simulink library "CreeksideLibrary030"  (R2016b)
settings: Solver=VariableStepAuto  StartTime=0.0  StopTime=10.0  RelTol=1e-3  EnableMultiTasking=on
libraries: simulink x4
settings Model: Creator=Jared  LastModifiedBy=Ika
settings DataIOCC: LimitDataPoints=on
settings OptimizationCC: LifeSpan=inf
settings DebuggingCC: AllowSymbolicDim=off  SFUnexpectedBacktrackingDiag=warning  SFNoUnconditionalDefaultTransitionDiag=warning  SFExecutionAtInitializationDiag=none
settings ModelReferenceCC: PropagateSignalLabelsOutOfModel=off
settings GRTTargetCC: TargetLangStandard=C89/C90 (ANSI)
settings ConfigComp: CovMetricSettings=dw  CovHtmlReporting=on  CovSaveCumulativeToWorkspaceVar=on  CovSaveSingleToWorkspaceVar=on  CovExternalEMLEnable=off

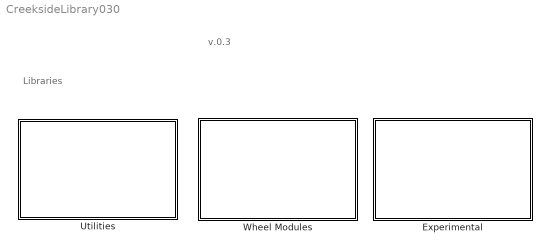
== system CreeksideLibrary030 ==
  note: Libraries
  note: v.0.3
  Experimental : Subsystem
      mask Display: image('gearBlock.png');
  Utilities : Subsystem
      mask Display: image('utilities.png');
  Wheel Modules : Subsystem
      mask Display: image('gearBlock.png');

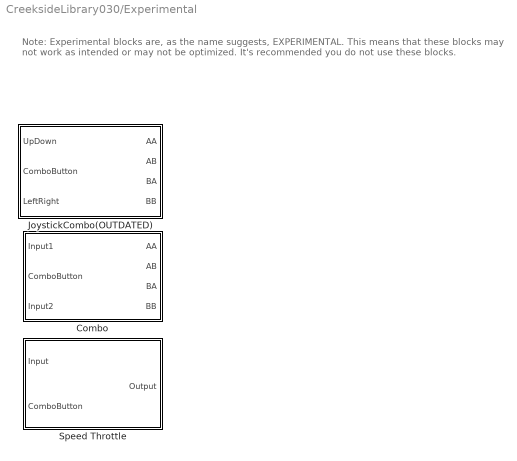
== system CreeksideLibrary030/Experimental ==
  note: Note: Experimental blocks are, as the name suggests, EXPERIMENTAL.
      | This means that these blocks may not work as intended or may not be optimized.
      | It's recommended you do not use these blocks.
  Combo : Subsystem  mask(Joystick Combo v.0.2.1){AAGain=1, ABGain=1, BAGain=1, BBGain=1}
      mask prompts: AAGain "AA value multiplier"; ABGain "AB value multiplier"; BAGain "BA value multiplier"; BBGain "BB value multiplier"
      mask help:
      | WARNING: Experimental version of Combo. This will have limited
      | functionality and may be buggy.
      |
      | Allows you to control multiple blocks using a joystick and a button.
      |
      | Link vertical joystick channels to UpDown, link horizontal joystick
      | channels LeftRight, and link a button to ComboButton.
      |
      | AA = Up/Down while not holding combo
      | AB = Left/Right while not holding combo
      | BA = Up/Down while holding combo
      | BB = Left/Right while holding combo
      mask Display:
      | pic = imread('globeMotor.png');
      | image(pic,[0.25 0.2 0.5 0.5]);
      | color('blue');
      | text(1,1,'CT','horizontalAlignment','right','verticalAlignment','top');
  JoystickCombo(OUTDATED) : MATLAB Function  TreatAsAtomicUnit=on  mask(Joystick Combo v.0.1.1){ButtonJoystick=off}
      mask prompts: ButtonJoystick "Using buttons?"
      mask help:
      | WARNING: Experimental version of Combo. This will have limited
      | functionality and may be buggy. Parameters have no effect on the block.
      |
      | Allows you to control multiple blocks using a joystick and a button.
      | Link vertical joystick channels to UpDown, link horizontal joystick
      | channels LeftRight, and link a button to ComboButton.
      |
      | AA = Up/Down while not holding combo
      | AB = Left/Right while not holding combo
      | BA = Up/Down while holding combo
      | BB = Left/Right while holding combo
  Speed Throttle : Subsystem  AncestorBlock=CreeksideLibraryExperimental023/Experimental/Combo  mask(Speed Throttle){}
      mask help:
      | (This is stable, just unoptimized. It's fine to use this block.)
      | While holding down a specific button, throttle the input speed.
      mask Display:
      | pic = imread('globeMotor.png');
      | image(pic,[0.25 0.2 0.5 0.5]);
      | color('blue');
      | text(1,1,'CT','horizontalAlignment','right','verticalAlignment','top');

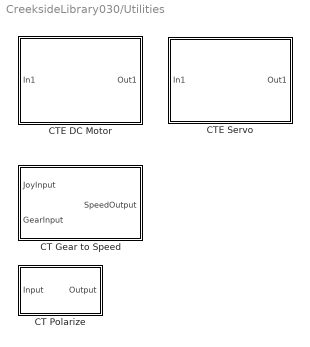
== system CreeksideLibrary030/Utilities ==
  CT Gear to Speed : Subsystem  mask(CT Gear to Speed){gearFourSpeed=1, gearThreeSpeed=0.5, gearTwoSpeed=-0.5, gearOneSpeed=-1}
      mask prompts: gearFourSpeed "Gear Four"; gearThreeSpeed "Gear Three"; gearTwoSpeed "Gear Two"; gearOneSpeed "Gear One"
      mask help:
      | This block finds the gear input and, depending on the set gear multipliers, multiplies the joystick input.
      | Gear four is the default speed.
      mask Display:
      | color('blue');
      | text(1,1,'CT','horizontalAlignment','right','verticalAlignment','top');
  CT Polarize : MATLAB Function  TreatAsAtomicUnit=on  mask(CT Convert 1/0 to -1/1){}
      mask help: When the input to this block is 1, the output is -1. When the input to this block is 0, the output is 1.
      settings: CopyFcn=set_param(gcb, 'LinkStatus', 'none') ;
  CTE DC Motor : Subsystem  mask(CTE DC Motor){motor=1, scaleFactor=1/13.5, lowSaturation=-127, highSaturation=127, SimulationOut=on}
      mask prompts: motor "Motor Channel"; scaleFactor "Gearing Ratio"; lowSaturation "Lowest input value"; highSaturation "Highest input value"; SimulationOut "Simulation output port?"
      mask help: Modified version of the VEX DC Motor block. This block has extra functionality and is more flexible. Motor Channel sets the port that the gain will be applied to. Gearing Ratio sets the number that the speed output will be modified by. Lowest input value controls the lowest input that will be applied to the motor. Highest input value controls the highest input that will be applied to the motor. If you're new to Simulink, it's recommended that you use the VEX DC Motor rather than this.
      mask init:
      | md = 'image(''GlobeMotor.png'',[0.07 0.2 0.77 0.65] );';
      | if ~SimulationOut
      |     replace_block(gcb, 'FollowLinks', 'on', 'BlockType', 'Outport', 'Terminator','noprompt');
      | else
      |     replace_block(gcb, 'FollowLinks', 'on', 'BlockType', 'Terminator','Outport', 'noprompt');
      | end
      | md =   [md,10,...
      |         'text(.5,.15,[''Port:'',motor], ''horizontalAlignment'', ''center'')',10,...
      |         'color(''blue'');',10,...
      |         'text(1,1,''CT'',''horizontalAlignment'',''right'',''verticalAlignment'',''top'');'];
      | set_param(gcb, 'MaskDisplay', md);
      mask TypeOptions motor: 1 | 2 | 3 | 4 | 5 | 6 | 7 | 8 | 9 | 10
      mask Display:
      | image('GlobeMotor.png',[0.07 0.2 0.77 0.65] );
      | text(.5,.15,['Port:',motor], 'horizontalAlignment', 'center')
      | color('blue');
      | text(1,1,'CT','horizontalAlignment','right','verticalAlignment','top');
  CTE Servo : Subsystem  mask(CTE Servo Motor){motor=1, scaleFactor=60/127, lowSaturation=-127, highSaturation=127, SimulationOut=on}
      mask prompts: motor "Motor Channel"; scaleFactor "Gearing Ratio"; lowSaturation "Lowest input value"; highSaturation "Highest input value"; SimulationOut "Simulation output port?"
      mask help:
      | (May be broken, take caution when using this block and consider using the default VEX Servo block.)
      | Modified version of the VEX Servo Motor block. This block has extra functionality and is more flexible. Motor Channel sets the port that the gain will be applied to. Gearing Ratio sets the number that the speed output will be modified by. Lowest input value controls the lowest input that will be applied to the servo. Highest input value controls the highest input that will be applied to the servo. If you're new to Simulink, it's recommended that you use the VEX Servo Motor rather than this.
      mask init:
      | md = 'image(''ServoMotor.png'',[0.07 0.2 0.77 0.65] );';
      | if ~SimulationOut
      |     replace_block(gcb, 'FollowLinks', 'on', 'BlockType', 'Outport', 'Terminator','noprompt');
      | else
      |     replace_block(gcb, 'FollowLinks', 'on', 'BlockType', 'Terminator','Outport', 'noprompt');
      | end
      | md =   [md,10,...
      |         'text(.5,.15,[''Port:'',motor], ''horizontalAlignment'', ''center'')',10,...
      |         'color(''blue'');',10,...
      |         'text(1,1,''CT'',''horizontalAlignment'',''right'',''verticalAlignment'',''top'');'];
      | set_param(gcb, 'MaskDisplay', md);
      mask TypeOptions motor: 1 | 2 | 3 | 4 | 5 | 6 | 7 | 8 | 9 | 10
      mask Display:
      | image('ServoMotor.png',[0.07 0.2 0.77 0.65] );
      | text(.5,.15,['Port:',motor], 'horizontalAlignment', 'center')
      | color('blue');
      | text(1,1,'CT','horizontalAlignment','right','verticalAlignment','top');

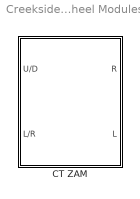
== system CreeksideLibrary030/Wheel Modules ==
  CT ZAM : Subsystem  AncestorBlock=CreeksideLibraryExperimental023/Wheel Modules/CT ZTBAModule  mask(Zero-Turn Based Arcade Module){}
      mask help: This block allows you to easily make a functional robot with zero-turn capabilities, curving capabilities, and easy driving while only using one stick.
      mask Display:
      | pic = imread('arcadeModule.png');
      | image(pic,[0.25 0.2 0.5 0.5]);
      | color('blue');
      | text(1,1,'CT','horizontalAlignment','right','verticalAlignment','top');

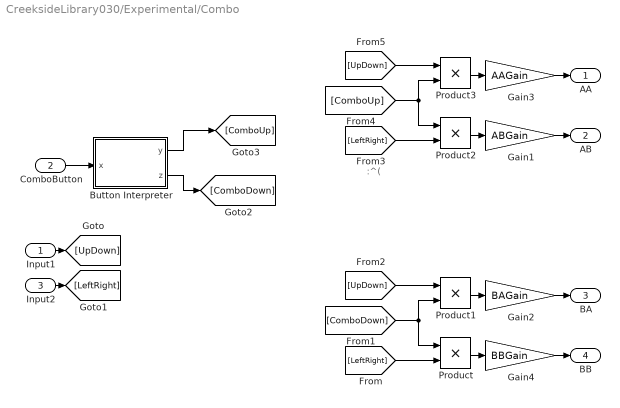
== system CreeksideLibrary030/Experimental/Combo ==
  note: :^(
  Input1 : Inport
  ComboButton : Inport  Port=2
  Input2 : Inport  Port=3
  Button Interpreter : MATLAB Function  TreatAsAtomicUnit=on  mask(Function){}
      mask help: Fixes the ComboButton input from going crazy
  Gain1 : Gain  Gain=ABGain
  Gain2 : Gain  Gain=BAGain
  Gain3 : Gain  Gain=AAGain
  Gain4 : Gain  Gain=BBGain
  Product{,1..3} (4 alike) : Product  RndMeth=Zero
  AA : Outport
  AB : Outport  Port=2
  BA : Outport  Port=3
  BB : Outport  Port=4
  wires:
  Input1/1 -> [UpDown]
  Input2/1 -> [LeftRight]
  [LeftRight] -> Product/2
  [ComboDown] -> Product/1, Product1/2
  [UpDown] -> Product1/1
  [LeftRight] -> Product2/2
  [ComboUp] -> Product2/1, Product3/2
  [UpDown] -> Product3/1
  ComboButton/1 -> Button Interpreter/1(x)
  Button Interpreter/1(y) -> [ComboUp]
  Button Interpreter/2(z) -> [ComboDown]
  Product3/1 -> Gain3/1
  Gain3/1 -> AA/1
  Product2/1 -> Gain1/1
  Gain1/1 -> AB/1
  Gain2/1 -> BA/1
  Gain4/1 -> BB/1
  Product1/1 -> Gain2/1
  Product/1 -> Gain4/1

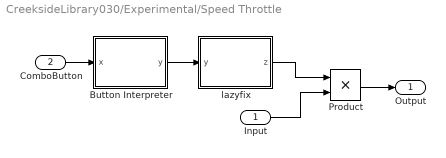
== system CreeksideLibrary030/Experimental/Speed Throttle ==
  Input : Inport
  ComboButton : Inport  Port=2
  Button Interpreter : MATLAB Function  TreatAsAtomicUnit=on  mask(Function){}
      mask help: Fixes the ComboButton input from going crazy
  Product : Product
  lazyfix : MATLAB Function  TreatAsAtomicUnit=on  mask(Function){}
      mask help: Fixes the ComboButton input from going crazy
  Output : Outport
  wires:
  ComboButton/1 -> Button Interpreter/1(x)
  Button Interpreter/1(y) -> lazyfix/1(y)
  lazyfix/1(z) -> Product/1
  Input/1 -> Product/2
  Product/1 -> Output/1

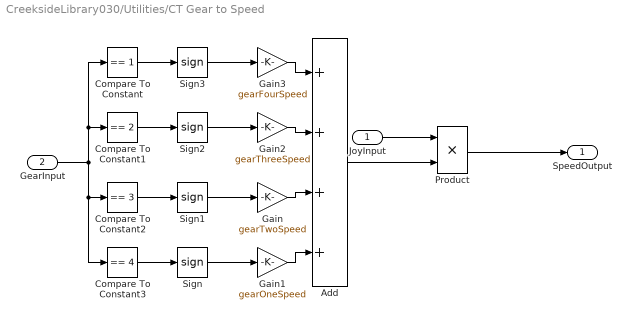
== system CreeksideLibrary030/Utilities/CT Gear to Speed ==
  JoyInput : Inport
  GearInput : Inport  Port=2
  Add : Sum  Inputs=++++
  Compare To Constant : simulink/Logic and Bit Operations/Compare To Constant  relop===  const=1  OutDataTypeStr=boolean
  Compare To Constant1 : simulink/Logic and Bit Operations/Compare To Constant  relop===  const=2  OutDataTypeStr=boolean
  Compare To Constant2 : simulink/Logic and Bit Operations/Compare To Constant  relop===  const=3  OutDataTypeStr=boolean
  Compare To Constant3 : simulink/Logic and Bit Operations/Compare To Constant  relop===  const=4  OutDataTypeStr=boolean
  Gain : Gain  Gain=gearTwoSpeed
  Gain1 : Gain  Gain=gearOneSpeed
  Gain2 : Gain  Gain=gearThreeSpeed
  Gain3 : Gain  Gain=gearFourSpeed
  Product : Product  RndMeth=Zero
  Sign{,1..3} (4 alike) : Signum
  SpeedOutput : Outport
  wires:
  Compare To Constant/1 -> Sign3/1
  Sign1/1 -> Gain/1
  Compare To Constant3/1 -> Sign/1
  Compare To Constant1/1 -> Sign2/1
  Add/1 -> Product/2
  Sign/1 -> Gain1/1
  JoyInput/1 -> Product/1
  Sign3/1 -> Gain3/1
  Gain2/1 -> Add/2
  Gain3/1 -> Add/1
  Compare To Constant2/1 -> Sign1/1
  Sign2/1 -> Gain2/1
  Product/1 -> SpeedOutput/1
  Gain1/1 -> Add/4
  GearInput/1 -> Compare To Constant3/1, Compare To Constant2/1, Compare To Constant1/1, Compare To Constant/1
  Gain/1 -> Add/3

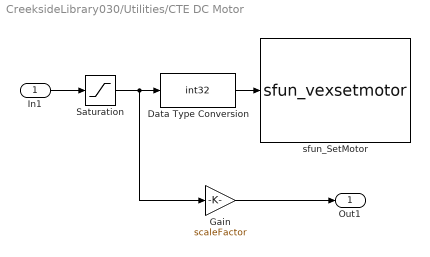
== system CreeksideLibrary030/Utilities/CTE DC Motor ==
  In1 : Inport
  Data Type Conversion : DataTypeConversion  OutDataTypeStr=int32  RndMeth=Round
  Gain : Gain  Gain=scaleFactor  OutDataTypeStr=Inherit: Same as input
  Saturation : Saturate  UpperLimit=highSaturation  LowerLimit=lowSaturation
  sfun_SetMotor : S-Function  FunctionName=sfun_vexsetmotor  Parameters=motor  SFunctionDeploymentMode=off  EnableBusSupport=off
  Out1 : Outport
  wires:
  Data Type Conversion/1 -> sfun_SetMotor/1
  Saturation/1 -> Data Type Conversion/1, Gain/1
  Gain/1 -> Out1/1
  In1/1 -> Saturation/1

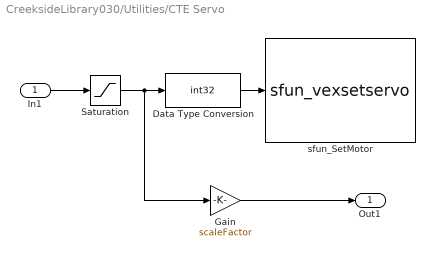
== system CreeksideLibrary030/Utilities/CTE Servo ==
  In1 : Inport
  Data Type Conversion : DataTypeConversion  OutDataTypeStr=int32  RndMeth=Round
  Gain : Gain  Gain=scaleFactor  OutDataTypeStr=Inherit: Same as input
  Saturation : Saturate  UpperLimit=highSaturation  LowerLimit=lowSaturation
  sfun_SetMotor : S-Function  FunctionName=sfun_vexsetservo  Parameters=motor  SFunctionDeploymentMode=off  EnableBusSupport=off
  Out1 : Outport
  wires:
  In1/1 -> Saturation/1
  Data Type Conversion/1 -> sfun_SetMotor/1
  Gain/1 -> Out1/1
  Saturation/1 -> Gain/1, Data Type Conversion/1

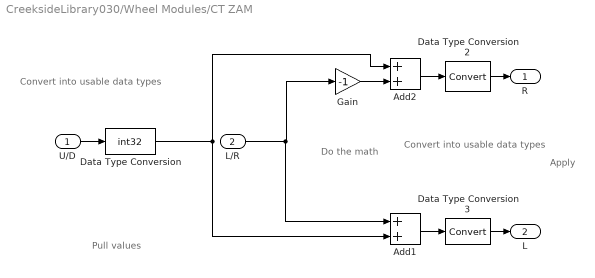
== system CreeksideLibrary030/Wheel Modules/CT ZAM ==
  note: Do the math
  note: Pull values
  note: Convert into usable data types
  note: Convert into usable
      | data types
  note: Apply
  U/D : Inport
  L/R : Inport  Port=2
  Add1 : Sum
  Add2 : Sum
  Data Type Conversion : DataTypeConversion  OutDataTypeStr=int32
  Data Type Conversion2 : DataTypeConversion
  Data Type Conversion3 : DataTypeConversion
  Gain : Gain  Gain=-1
  R : Outport
  L : Outport  Port=2
  wires:
  Add2/1 -> Data Type Conversion2/1
  Add1/1 -> Data Type Conversion3/1
  Data Type Conversion2/1 -> R/1
  Data Type Conversion3/1 -> L/1
  L/R/1 -> Add1/1, Gain/1
  Data Type Conversion/1 -> Add2/1, Add1/2
  U/D/1 -> Data Type Conversion/1
  Gain/1 -> Add2/2

== matlab function CreeksideLibrary030/Experimental/Speed Throttle/Button Interpreter ==
  data: x input; y output
function y  = fcn(x)
%#codegen
if x==0
    y=0;
else
    y=1;
end

== matlab function CreeksideLibrary030/Experimental/Combo/Button Interpreter ==
  data: x input; y output; z output
function [y,z] = fcn(x)
%#codegen
if x==0
    y=1;
    z=0;
else
    y=0;
    z=1;
end

== matlab function CreeksideLibrary030/Experimental/JoystickCombo(OUTDATED) ==
  data: AA output; AB output; BA output; UpDown input; ComboButton input; LeftRight input; BB output
function [AA,AB,BA,BB]= fcn(UpDown,ComboButton,LeftRight)
%#codegen
if ComboButton==0
    AA=UpDown
    AB=LeftRight
    BA=0
    BB=0
else
    AA=0
    AB=0
    BA=UpDown
    BB=LeftRight
end

== matlab function CreeksideLibrary030/Experimental/Speed Throttle/lazyfix ==
  data: y input; z output
function z = fcn(y)
%#codegen
if y==0
    z=1;
else
    z=.5;
end

== matlab function CreeksideLibrary030/Utilities/CT Polarize ==
  data: Input input; Output output
function Output = fcn(Input)
    %#codegen
    x=0-2;
    Output=Input*x+1;
